simulink model "test1"  (R2020a)
settings: Solver=VariableStepAuto  StartTime=0.0  StopTime=inf  FixedStep=Ts  RelTol=1e-3
PostLoadFcn:
  | , if any(exist('dsrtsu_mdlpostloadfcn', 'file') ~= 0), dsrtsu_mdlpostloadfcn('Execute', bdroot); end,
InitFcn:
  | , if any(exist('rtifpga_mdlclblib', 'file') ~= 0), rtifpga_mdlclblib('Init', bdroot); end,
model workspace (MAT data in the model file):
  FPGA_test1_1_Interrupt_1_1_write : Simulink.Signal (value not decoded)
  FPGA_test1_1_Register_1_1_1_write : Simulink.Signal (value not decoded)
  FPGA_test1_1_Register_2_1_1_write : Simulink.Signal (value not decoded)
  FPGA_test1_1_Register_3_1_1_write : Simulink.Signal (value not decoded)
  FPGA_test1_1_Register_4_1_1_write : Simulink.Signal (value not decoded)
values from neighbouring files (symbols this model uses):
  clamp_threshold = 200    [param.m]
  io_fixed_gain = 10*1000/(3*100)    (= 33.3333333333)    [param.m]
  io_sonda_gain = 10/0.010    (= 1000)    [param.m]
  ioa_gain = 1    [param.m]
  ioa_offset = 0.12    [param.m]
  iob_gain = 1    [param.m]
  iob_offset = 0.06    [param.m]
  ioc_gain = 1    [param.m]
  ioc_offset = -0.1    [param.m]
  Ts = 20e-6    (= 2e-05)    [param.m]
  vclamp_gain = 1010    [param.m]
  vclamp_offset = 10.5    [param.m]
  vi_fixed_gain = 10*44    (= 440)    [param.m]
  vi_sonda_gain = 10*200    (= 2000)    [param.m]
  via_gain = 1    [param.m]
  via_offset = 2.2    [param.m]
  vib_gain = 1    [param.m]
  vib_offset = 3    [param.m]
  vic_gain = 1    [param.m]
  vic_offset = 4.2    [param.m]
libraries: xbsIndex_r4 x428, rti1202lib_adc_class1 x9, rtiproclib x6, simulink x2, rtifpgainterfacelib x1
(part 7 of 7)

== system test1/4_step/FPGA_IO_WRITE_BL6/dig_inout_tp1 ==
  note: The nominal input range is NOT simulated because
      | the HW does not saturate according to the input range.
  note: The Digital In value is simulated by Threshold voltage detection.
  data_in_i : Inport
  enable_i : Inport  Port=2
  data_out_i : Inport  Port=3
  direction_i : Inport  Port=4
  Data Type Conversion : DataTypeConversion
  Data Type Conversion1 : DataTypeConversion
  Disabled Input Value : Constant  Value=0
  Disabled Output Value : Constant  Value=0
  Invert : Constant  Value=inverted_dio
  Invert1 : Constant  Value=inverted_dio
  Inverter : Logic  Operator=NOT  AllPortsSameDT=off  OutDataTypeStr=boolean
  Inverter1 : Logic  AllPortsSameDT=off  OutDataTypeStr=boolean
  Inverter2 : Logic  Operator=NOT  AllPortsSameDT=off  OutDataTypeStr=boolean
  Inverter3 : Logic  AllPortsSameDT=off  OutDataTypeStr=boolean
  Inverter4 : Logic  Operator=NOT  AllPortsSameDT=off  OutDataTypeStr=boolean
  Relational Operator : RelationalOperator  OutDataTypeStr=boolean  RndMeth=Nearest
  Switch{,1..3} (4 alike) : Switch  Threshold=1
  Threshold Voltage : Constant  Value=2
  Voltage : Gain  Gain=voltage  ParamDataTypeStr=float('double')
  data_in_o : Outport  VectorParamsAs1DForOutWhenUnconnected=off
  data_out_o : Outport  Port=2  VectorParamsAs1DForOutWhenUnconnected=off
  wires:
  Voltage/1 -> data_out_o/1
  Data Type Conversion1/1 -> Inverter3/2, Inverter2/1
  Data Type Conversion/1 -> Inverter3/1, Inverter1/1
  Switch3/1 -> Voltage/1
  Switch2/1 -> Switch3/3, Inverter4/1
  Inverter4/1 -> Switch3/1
  Invert1/1 -> Switch3/2
  data_out_i/1 -> Switch2/1
  Inverter3/1 -> Switch2/2
  Disabled Output Value/1 -> Switch2/3
  Inverter2/1 -> Inverter1/2
  direction_i/1 -> Data Type Conversion1/1
  Inverter1/1 -> Switch/2
  enable_i/1 -> Data Type Conversion/1
  Switch/1 -> Switch1/3, Inverter/1
  Relational Operator/1 -> Switch/1
  Inverter/1 -> Switch1/1
  Invert/1 -> Switch1/2
  Switch1/1 -> data_in_o/1
  Disabled Input Value/1 -> Switch/3
  Threshold Voltage/1 -> Relational Operator/2
  data_in_i/1 -> Relational Operator/1

== system test1/4_step/FPGA_IO_WRITE_BL7/dig_inout_tp1 ==
  note: The nominal input range is NOT simulated because
      | the HW does not saturate according to the input range.
  note: The Digital In value is simulated by Threshold voltage detection.
  data_in_i : Inport
  enable_i : Inport  Port=2
  data_out_i : Inport  Port=3
  direction_i : Inport  Port=4
  Data Type Conversion : DataTypeConversion
  Data Type Conversion1 : DataTypeConversion
  Disabled Input Value : Constant  Value=0
  Disabled Output Value : Constant  Value=0
  Invert : Constant  Value=inverted_dio
  Invert1 : Constant  Value=inverted_dio
  Inverter : Logic  Operator=NOT  AllPortsSameDT=off  OutDataTypeStr=boolean
  Inverter1 : Logic  AllPortsSameDT=off  OutDataTypeStr=boolean
  Inverter2 : Logic  Operator=NOT  AllPortsSameDT=off  OutDataTypeStr=boolean
  Inverter3 : Logic  AllPortsSameDT=off  OutDataTypeStr=boolean
  Inverter4 : Logic  Operator=NOT  AllPortsSameDT=off  OutDataTypeStr=boolean
  Relational Operator : RelationalOperator  OutDataTypeStr=boolean  RndMeth=Nearest
  Switch{,1..3} (4 alike) : Switch  Threshold=1
  Threshold Voltage : Constant  Value=2
  Voltage : Gain  Gain=voltage  ParamDataTypeStr=float('double')
  data_in_o : Outport  VectorParamsAs1DForOutWhenUnconnected=off
  data_out_o : Outport  Port=2  VectorParamsAs1DForOutWhenUnconnected=off
  wires:
  Voltage/1 -> data_out_o/1
  Data Type Conversion1/1 -> Inverter3/2, Inverter2/1
  Data Type Conversion/1 -> Inverter3/1, Inverter1/1
  Switch3/1 -> Voltage/1
  Switch2/1 -> Switch3/3, Inverter4/1
  Inverter4/1 -> Switch3/1
  Invert1/1 -> Switch3/2
  data_out_i/1 -> Switch2/1
  Inverter3/1 -> Switch2/2
  Disabled Output Value/1 -> Switch2/3
  Inverter2/1 -> Inverter1/2
  direction_i/1 -> Data Type Conversion1/1
  Inverter1/1 -> Switch/2
  enable_i/1 -> Data Type Conversion/1
  Switch/1 -> Switch1/3, Inverter/1
  Relational Operator/1 -> Switch/1
  Inverter/1 -> Switch1/1
  Invert/1 -> Switch1/2
  Switch1/1 -> data_in_o/1
  Disabled Input Value/1 -> Switch/3
  Threshold Voltage/1 -> Relational Operator/2
  data_in_i/1 -> Relational Operator/1

== system test1/4_step/FPGA_IO_WRITE_BL8/dig_inout_tp1 ==
  note: The nominal input range is NOT simulated because
      | the HW does not saturate according to the input range.
  note: The Digital In value is simulated by Threshold voltage detection.
  data_in_i : Inport
  enable_i : Inport  Port=2
  data_out_i : Inport  Port=3
  direction_i : Inport  Port=4
  Data Type Conversion : DataTypeConversion
  Data Type Conversion1 : DataTypeConversion
  Disabled Input Value : Constant  Value=0
  Disabled Output Value : Constant  Value=0
  Invert : Constant  Value=inverted_dio
  Invert1 : Constant  Value=inverted_dio
  Inverter : Logic  Operator=NOT  AllPortsSameDT=off  OutDataTypeStr=boolean
  Inverter1 : Logic  AllPortsSameDT=off  OutDataTypeStr=boolean
  Inverter2 : Logic  Operator=NOT  AllPortsSameDT=off  OutDataTypeStr=boolean
  Inverter3 : Logic  AllPortsSameDT=off  OutDataTypeStr=boolean
  Inverter4 : Logic  Operator=NOT  AllPortsSameDT=off  OutDataTypeStr=boolean
  Relational Operator : RelationalOperator  OutDataTypeStr=boolean  RndMeth=Nearest
  Switch{,1..3} (4 alike) : Switch  Threshold=1
  Threshold Voltage : Constant  Value=2
  Voltage : Gain  Gain=voltage  ParamDataTypeStr=float('double')
  data_in_o : Outport  VectorParamsAs1DForOutWhenUnconnected=off
  data_out_o : Outport  Port=2  VectorParamsAs1DForOutWhenUnconnected=off
  wires:
  Voltage/1 -> data_out_o/1
  Data Type Conversion1/1 -> Inverter3/2, Inverter2/1
  Data Type Conversion/1 -> Inverter3/1, Inverter1/1
  Switch3/1 -> Voltage/1
  Switch2/1 -> Switch3/3, Inverter4/1
  Inverter4/1 -> Switch3/1
  Invert1/1 -> Switch3/2
  data_out_i/1 -> Switch2/1
  Inverter3/1 -> Switch2/2
  Disabled Output Value/1 -> Switch2/3
  Inverter2/1 -> Inverter1/2
  direction_i/1 -> Data Type Conversion1/1
  Inverter1/1 -> Switch/2
  enable_i/1 -> Data Type Conversion/1
  Switch/1 -> Switch1/3, Inverter/1
  Relational Operator/1 -> Switch/1
  Inverter/1 -> Switch1/1
  Invert/1 -> Switch1/2
  Switch1/1 -> data_in_o/1
  Disabled Input Value/1 -> Switch/3
  Threshold Voltage/1 -> Relational Operator/2
  data_in_i/1 -> Relational Operator/1

== system test1/4_step/FPGA_IO_WRITE_BL9/dig_inout_tp1 ==
  note: The nominal input range is NOT simulated because
      | the HW does not saturate according to the input range.
  note: The Digital In value is simulated by Threshold voltage detection.
  data_in_i : Inport
  enable_i : Inport  Port=2
  data_out_i : Inport  Port=3
  direction_i : Inport  Port=4
  Data Type Conversion : DataTypeConversion
  Data Type Conversion1 : DataTypeConversion
  Disabled Input Value : Constant  Value=0
  Disabled Output Value : Constant  Value=0
  Invert : Constant  Value=inverted_dio
  Invert1 : Constant  Value=inverted_dio
  Inverter : Logic  Operator=NOT  AllPortsSameDT=off  OutDataTypeStr=boolean
  Inverter1 : Logic  AllPortsSameDT=off  OutDataTypeStr=boolean
  Inverter2 : Logic  Operator=NOT  AllPortsSameDT=off  OutDataTypeStr=boolean
  Inverter3 : Logic  AllPortsSameDT=off  OutDataTypeStr=boolean
  Inverter4 : Logic  Operator=NOT  AllPortsSameDT=off  OutDataTypeStr=boolean
  Relational Operator : RelationalOperator  OutDataTypeStr=boolean  RndMeth=Nearest
  Switch{,1..3} (4 alike) : Switch  Threshold=1
  Threshold Voltage : Constant  Value=2
  Voltage : Gain  Gain=voltage  ParamDataTypeStr=float('double')
  data_in_o : Outport  VectorParamsAs1DForOutWhenUnconnected=off
  data_out_o : Outport  Port=2  VectorParamsAs1DForOutWhenUnconnected=off
  wires:
  Voltage/1 -> data_out_o/1
  Data Type Conversion1/1 -> Inverter3/2, Inverter2/1
  Data Type Conversion/1 -> Inverter3/1, Inverter1/1
  Switch3/1 -> Voltage/1
  Switch2/1 -> Switch3/3, Inverter4/1
  Inverter4/1 -> Switch3/1
  Invert1/1 -> Switch3/2
  data_out_i/1 -> Switch2/1
  Inverter3/1 -> Switch2/2
  Disabled Output Value/1 -> Switch2/3
  Inverter2/1 -> Inverter1/2
  direction_i/1 -> Data Type Conversion1/1
  Inverter1/1 -> Switch/2
  enable_i/1 -> Data Type Conversion/1
  Switch/1 -> Switch1/3, Inverter/1
  Relational Operator/1 -> Switch/1
  Inverter/1 -> Switch1/1
  Invert/1 -> Switch1/2
  Switch1/1 -> data_in_o/1
  Disabled Input Value/1 -> Switch/3
  Threshold Voltage/1 -> Relational Operator/2
  data_in_i/1 -> Relational Operator/1

== system test1/4_step/FPGA_XDATA_READ_BL1/phs_read_register ==
  note: Subsystem simulating the phs bus
      | access via RTLib functions.
  note: Subsystem simulating the communication
      | function specific behaviour. This is how the
      | FPGA framework driver takes effect on the data.
  data_i : Inport
  com_fct_model : Subsystem
  phs/rtlib_sim_model : Subsystem
  data_o : Outport  VectorParamsAs1DForOutWhenUnconnected=off
  data_new_o : Outport  Port=2  VectorParamsAs1DForOutWhenUnconnected=off
  wires:
  com_fct_model/2(data_new_o) -> data_new_o/1
  phs/rtlib_sim_model/1(data_o1) -> com_fct_model/1(data_i1)
  com_fct_model/1(data_o1) -> data_o/1
  data_i/1 -> phs/rtlib_sim_model/1(data_i1)

== system test1/4_step/FPGA_XDATA_READ_BL2/phs_read_register ==
  note: Subsystem simulating the phs bus
      | access via RTLib functions.
  note: Subsystem simulating the communication
      | function specific behaviour. This is how the
      | FPGA framework driver takes effect on the data.
  data_i : Inport
  com_fct_model : Subsystem
  phs/rtlib_sim_model : Subsystem
  data_o : Outport  VectorParamsAs1DForOutWhenUnconnected=off
  data_new_o : Outport  Port=2  VectorParamsAs1DForOutWhenUnconnected=off
  wires:
  com_fct_model/2(data_new_o) -> data_new_o/1
  phs/rtlib_sim_model/1(data_o1) -> com_fct_model/1(data_i1)
  com_fct_model/1(data_o1) -> data_o/1
  data_i/1 -> phs/rtlib_sim_model/1(data_i1)

== system test1/4_step/FPGA_XDATA_READ_BL3/phs_read_register ==
  note: Subsystem simulating the phs bus
      | access via RTLib functions.
  note: Subsystem simulating the communication
      | function specific behaviour. This is how the
      | FPGA framework driver takes effect on the data.
  data_i : Inport
  com_fct_model : Subsystem
  phs/rtlib_sim_model : Subsystem
  data_o : Outport  VectorParamsAs1DForOutWhenUnconnected=off
  data_new_o : Outport  Port=2  VectorParamsAs1DForOutWhenUnconnected=off
  wires:
  com_fct_model/2(data_new_o) -> data_new_o/1
  phs/rtlib_sim_model/1(data_o1) -> com_fct_model/1(data_i1)
  com_fct_model/1(data_o1) -> data_o/1
  data_i/1 -> phs/rtlib_sim_model/1(data_i1)

== system test1/4_step/FPGA_XDATA_READ_BL4/phs_read_register ==
  note: Subsystem simulating the phs bus
      | access via RTLib functions.
  note: Subsystem simulating the communication
      | function specific behaviour. This is how the
      | FPGA framework driver takes effect on the data.
  data_i : Inport
  com_fct_model : Subsystem
  phs/rtlib_sim_model : Subsystem
  data_o : Outport  VectorParamsAs1DForOutWhenUnconnected=off
  data_new_o : Outport  Port=2  VectorParamsAs1DForOutWhenUnconnected=off
  wires:
  com_fct_model/2(data_new_o) -> data_new_o/1
  phs/rtlib_sim_model/1(data_o1) -> com_fct_model/1(data_i1)
  com_fct_model/1(data_o1) -> data_o/1
  data_i/1 -> phs/rtlib_sim_model/1(data_i1)

== system test1/RTI Data/RTI Data Store/RTI Data Store ==
  RTI Data Store : Subsystem  mask(RTI_DATA_STORE){}
      mask help:
      | RTI Data Store Block. This block is used by RTI to store internal model dependent data. Deleting this block will result in data loss.
      |
      | NEVER DELETE, COPY, OR MODIFY THIS BLOCK!
      mask Help:
      | RTI Data Store Block. This block is used by RTI to store internal model dependent data. Deleting this block will result in data loss.
      | 
      | NEVER DELETE, COPY, OR MODIFY THIS BLOCK!
      mask Display: text(0.5, 0.5, ' ', 'HorizontalAlignment', 'center');

== system test1/4_step/FPGA_INT_BL1/phs_interrupt/com_fct_model ==
  data_i1 : Inport
  data_o1 : Outport  VectorParamsAs1DForOutWhenUnconnected=off
  wires:
  data_i1/1 -> data_o1/1

== system test1/4_step/FPGA_INT_BL1/phs_interrupt/phs//rtlib_sim_model ==
  note: - Detect the interrupt (rising edge).
      | - Generate function call.
  data_i1 : Inport
  Triggered Subsystem : Subsystem  TreatAsAtomicUnit=on
  data_o1 : Outport  VectorParamsAs1DForOutWhenUnconnected=off
  wires:
  Triggered Subsystem/1(Out1) -> data_o1/1
  data_i1/1 -> Triggered Subsystem/Trigger

== system test1/4_step/FPGA_XDATA_READ_BL1/phs_read_register/com_fct_model ==
  note: - Register data is presented to the FPGA application without data adaptions.
      |
      | - Register group accesses are implicitly simulated by simulink: all FPGA
      | communication function interface blocks are simulated within one task
      | with a unique sample time --> in- and ouputs are sampled simultaneously
      | and therefore data consistency is guaranteed.
  data_i1 : Inport
  Data_New_Calc : Subsystem
  Zero-Order Hold : ZeroOrderHold  SampleTime=fpga_sample_time
  data_o1 : Outport  VectorParamsAs1DForOutWhenUnconnected=off
  data_new_o : Outport  Port=2  VectorParamsAs1DForOutWhenUnconnected=off
  wires:
  Zero-Order Hold/1 -> data_o1/1
  Data_New_Calc/1(Out1) -> data_new_o/1
  data_i1/1 -> Zero-Order Hold/1, Data_New_Calc/1(In1)

== system test1/4_step/FPGA_XDATA_READ_BL1/phs_read_register/phs//rtlib_sim_model ==
  note: - The double to fixed-point conversion done by the XSG gateway behaves differently
      | than the conversion done by the RTLib C-code. Therefore the C-Code behaviour
      | is simulated via an s-function using the RTLib conversion technique including scaling and saturation.
  data_i1 : Inport
  S-Function : S-Function  FunctionName=DS1302_read_register  Parameters=mode;binaryPoint  SFunctionDeploymentMode=off  EnableBusSupport=off
  Zero-Order Hold : ZeroOrderHold  SampleTime=proc_sample_time
  data_o1 : Outport  VectorParamsAs1DForOutWhenUnconnected=off
  wires:
  Zero-Order Hold/1 -> S-Function/1
  S-Function/1 -> data_o1/1
  data_i1/1 -> Zero-Order Hold/1

== system test1/4_step/FPGA_XDATA_READ_BL2/phs_read_register/com_fct_model ==
  note: - Register data is presented to the FPGA application without data adaptions.
      |
      | - Register group accesses are implicitly simulated by simulink: all FPGA
      | communication function interface blocks are simulated within one task
      | with a unique sample time --> in- and ouputs are sampled simultaneously
      | and therefore data consistency is guaranteed.
  data_i1 : Inport
  Data_New_Calc : Subsystem
  Zero-Order Hold : ZeroOrderHold  SampleTime=fpga_sample_time
  data_o1 : Outport  VectorParamsAs1DForOutWhenUnconnected=off
  data_new_o : Outport  Port=2  VectorParamsAs1DForOutWhenUnconnected=off
  wires:
  Zero-Order Hold/1 -> data_o1/1
  Data_New_Calc/1(Out1) -> data_new_o/1
  data_i1/1 -> Zero-Order Hold/1, Data_New_Calc/1(In1)

== system test1/4_step/FPGA_XDATA_READ_BL2/phs_read_register/phs//rtlib_sim_model ==
  note: - The double to fixed-point conversion done by the XSG gateway behaves differently
      | than the conversion done by the RTLib C-code. Therefore the C-Code behaviour
      | is simulated via an s-function using the RTLib conversion technique including scaling and saturation.
  data_i1 : Inport
  S-Function : S-Function  FunctionName=DS1302_read_register  Parameters=mode;binaryPoint  SFunctionDeploymentMode=off  EnableBusSupport=off
  Zero-Order Hold : ZeroOrderHold  SampleTime=proc_sample_time
  data_o1 : Outport  VectorParamsAs1DForOutWhenUnconnected=off
  wires:
  Zero-Order Hold/1 -> S-Function/1
  S-Function/1 -> data_o1/1
  data_i1/1 -> Zero-Order Hold/1

== system test1/4_step/FPGA_XDATA_READ_BL3/phs_read_register/com_fct_model ==
  note: - Register data is presented to the FPGA application without data adaptions.
      |
      | - Register group accesses are implicitly simulated by simulink: all FPGA
      | communication function interface blocks are simulated within one task
      | with a unique sample time --> in- and ouputs are sampled simultaneously
      | and therefore data consistency is guaranteed.
  data_i1 : Inport
  Data_New_Calc : Subsystem
  Zero-Order Hold : ZeroOrderHold  SampleTime=fpga_sample_time
  data_o1 : Outport  VectorParamsAs1DForOutWhenUnconnected=off
  data_new_o : Outport  Port=2  VectorParamsAs1DForOutWhenUnconnected=off
  wires:
  Zero-Order Hold/1 -> data_o1/1
  Data_New_Calc/1(Out1) -> data_new_o/1
  data_i1/1 -> Zero-Order Hold/1, Data_New_Calc/1(In1)

== system test1/4_step/FPGA_XDATA_READ_BL3/phs_read_register/phs//rtlib_sim_model ==
  note: - The double to fixed-point conversion done by the XSG gateway behaves differently
      | than the conversion done by the RTLib C-code. Therefore the C-Code behaviour
      | is simulated via an s-function using the RTLib conversion technique including scaling and saturation.
  data_i1 : Inport
  S-Function : S-Function  FunctionName=DS1302_read_register  Parameters=mode;binaryPoint  SFunctionDeploymentMode=off  EnableBusSupport=off
  Zero-Order Hold : ZeroOrderHold  SampleTime=proc_sample_time
  data_o1 : Outport  VectorParamsAs1DForOutWhenUnconnected=off
  wires:
  Zero-Order Hold/1 -> S-Function/1
  S-Function/1 -> data_o1/1
  data_i1/1 -> Zero-Order Hold/1

== system test1/4_step/FPGA_XDATA_READ_BL4/phs_read_register/com_fct_model ==
  note: - Register data is presented to the FPGA application without data adaptions.
      |
      | - Register group accesses are implicitly simulated by simulink: all FPGA
      | communication function interface blocks are simulated within one task
      | with a unique sample time --> in- and ouputs are sampled simultaneously
      | and therefore data consistency is guaranteed.
  data_i1 : Inport
  Data_New_Calc : Subsystem
  Zero-Order Hold : ZeroOrderHold  SampleTime=fpga_sample_time
  data_o1 : Outport  VectorParamsAs1DForOutWhenUnconnected=off
  data_new_o : Outport  Port=2  VectorParamsAs1DForOutWhenUnconnected=off
  wires:
  Zero-Order Hold/1 -> data_o1/1
  Data_New_Calc/1(Out1) -> data_new_o/1
  data_i1/1 -> Zero-Order Hold/1, Data_New_Calc/1(In1)

== system test1/4_step/FPGA_XDATA_READ_BL4/phs_read_register/phs//rtlib_sim_model ==
  note: - The double to fixed-point conversion done by the XSG gateway behaves differently
      | than the conversion done by the RTLib C-code. Therefore the C-Code behaviour
      | is simulated via an s-function using the RTLib conversion technique including scaling and saturation.
  data_i1 : Inport
  S-Function : S-Function  FunctionName=DS1302_read_register  Parameters=mode;binaryPoint  SFunctionDeploymentMode=off  EnableBusSupport=off
  Zero-Order Hold : ZeroOrderHold  SampleTime=proc_sample_time
  data_o1 : Outport  VectorParamsAs1DForOutWhenUnconnected=off
  wires:
  Zero-Order Hold/1 -> S-Function/1
  S-Function/1 -> data_o1/1
  data_i1/1 -> Zero-Order Hold/1

== system test1/RTI Data/RTI Data Store/RTI Data Store/RTI Data Store ==
  RTI Data Store : Subsystem  mask(RTI_DATA_STORE){}
      mask help:
      | RTI Data Store Block. This block is used by RTI to store internal model dependent data. Deleting this block will result in data loss.
      |
      | NEVER DELETE, COPY, OR MODIFY THIS BLOCK!
      mask Help:
      | RTI Data Store Block. This block is used by RTI to store internal model dependent data. Deleting this block will result in data loss.
      | 
      | NEVER DELETE, COPY, OR MODIFY THIS BLOCK!
      mask Display: text(0.5, 0.5, ' ', 'HorizontalAlignment', 'center');

== system test1/4_step/FPGA_INT_BL1/phs_interrupt/phs//rtlib_sim_model/Triggered Subsystem ==
  Trigger : TriggerPort  VariantControl=(inherit)
  Function-Call Generator : simulink/Ports & Subsystems/Function-Call Generator  sample_time=-1  numberOfIterations=1
  Out1 : Outport  VectorParamsAs1DForOutWhenUnconnected=off
  wires:
  Function-Call Generator/1 -> Out1/1

== system test1/4_step/FPGA_XDATA_READ_BL1/phs_read_register/com_fct_model/Data_New_Calc ==
  note: The new data flag is presented whenever the input data port is sampled.
      | The flag is set to 1 for one FPGA simulation step and reset to 0 for the
      | remaining FPGA simulation steps contained within one processor simulation step.
  In1 : Inport
  Add : Sum
  Constant : Constant  Value=fpga_sample_time  SampleTime=fpga_sample_time
  Constant1 : Constant  Value=0
  Divide : Product  Inputs=*/
  Divide1 : Product  Inputs=*/
  Math Function : Math  Operator=mod  SignedPower=on  SaturateOnIntegerOverflow=on
  Relational Operator : RelationalOperator  Operator===  OutDataTypeStr=boolean  RndMeth=Nearest
  Unit Delay1 : UnitDelay  InitialCondition=-1  SampleTime=-1  HasFrameUpgradeWarning=on
  Weighted Sample Time1 : SampleTimeMath  TsampMathOp=Ts Only
  Out1 : Outport  VectorParamsAs1DForOutWhenUnconnected=off
  wires:
  Constant/1 -> Divide1/2, Divide1/1, Divide/2
  Weighted Sample Time1/1 -> Divide/1
  Math Function/1 -> Relational Operator/1
  Relational Operator/1 -> Out1/1
  In1/1 -> Weighted Sample Time1/1
  Divide1/1 -> Add/1
  Unit Delay1/1 -> Add/2
  Add/1 -> Unit Delay1/1, Math Function/1
  Constant1/1 -> Relational Operator/2
  Divide/1 -> Math Function/2

== system test1/4_step/FPGA_XDATA_READ_BL2/phs_read_register/com_fct_model/Data_New_Calc ==
  note: The new data flag is presented whenever the input data port is sampled.
      | The flag is set to 1 for one FPGA simulation step and reset to 0 for the
      | remaining FPGA simulation steps contained within one processor simulation step.
  In1 : Inport
  Add : Sum
  Constant : Constant  Value=fpga_sample_time  SampleTime=fpga_sample_time
  Constant1 : Constant  Value=0
  Divide : Product  Inputs=*/
  Divide1 : Product  Inputs=*/
  Math Function : Math  Operator=mod  SignedPower=on  SaturateOnIntegerOverflow=on
  Relational Operator : RelationalOperator  Operator===  OutDataTypeStr=boolean  RndMeth=Nearest
  Unit Delay1 : UnitDelay  InitialCondition=-1  SampleTime=-1  HasFrameUpgradeWarning=on
  Weighted Sample Time1 : SampleTimeMath  TsampMathOp=Ts Only
  Out1 : Outport  VectorParamsAs1DForOutWhenUnconnected=off
  wires:
  Constant/1 -> Divide1/2, Divide1/1, Divide/2
  Weighted Sample Time1/1 -> Divide/1
  Math Function/1 -> Relational Operator/1
  Relational Operator/1 -> Out1/1
  In1/1 -> Weighted Sample Time1/1
  Divide1/1 -> Add/1
  Unit Delay1/1 -> Add/2
  Add/1 -> Unit Delay1/1, Math Function/1
  Constant1/1 -> Relational Operator/2
  Divide/1 -> Math Function/2

== system test1/4_step/FPGA_XDATA_READ_BL3/phs_read_register/com_fct_model/Data_New_Calc ==
  note: The new data flag is presented whenever the input data port is sampled.
      | The flag is set to 1 for one FPGA simulation step and reset to 0 for the
      | remaining FPGA simulation steps contained within one processor simulation step.
  In1 : Inport
  Add : Sum
  Constant : Constant  Value=fpga_sample_time  SampleTime=fpga_sample_time
  Constant1 : Constant  Value=0
  Divide : Product  Inputs=*/
  Divide1 : Product  Inputs=*/
  Math Function : Math  Operator=mod  SignedPower=on  SaturateOnIntegerOverflow=on
  Relational Operator : RelationalOperator  Operator===  OutDataTypeStr=boolean  RndMeth=Nearest
  Unit Delay1 : UnitDelay  InitialCondition=-1  SampleTime=-1  HasFrameUpgradeWarning=on
  Weighted Sample Time1 : SampleTimeMath  TsampMathOp=Ts Only
  Out1 : Outport  VectorParamsAs1DForOutWhenUnconnected=off
  wires:
  Constant/1 -> Divide1/2, Divide1/1, Divide/2
  Weighted Sample Time1/1 -> Divide/1
  Math Function/1 -> Relational Operator/1
  Relational Operator/1 -> Out1/1
  In1/1 -> Weighted Sample Time1/1
  Divide1/1 -> Add/1
  Unit Delay1/1 -> Add/2
  Add/1 -> Unit Delay1/1, Math Function/1
  Constant1/1 -> Relational Operator/2
  Divide/1 -> Math Function/2

== system test1/4_step/FPGA_XDATA_READ_BL4/phs_read_register/com_fct_model/Data_New_Calc ==
  note: The new data flag is presented whenever the input data port is sampled.
      | The flag is set to 1 for one FPGA simulation step and reset to 0 for the
      | remaining FPGA simulation steps contained within one processor simulation step.
  In1 : Inport
  Add : Sum
  Constant : Constant  Value=fpga_sample_time  SampleTime=fpga_sample_time
  Constant1 : Constant  Value=0
  Divide : Product  Inputs=*/
  Divide1 : Product  Inputs=*/
  Math Function : Math  Operator=mod  SignedPower=on  SaturateOnIntegerOverflow=on
  Relational Operator : RelationalOperator  Operator===  OutDataTypeStr=boolean  RndMeth=Nearest
  Unit Delay1 : UnitDelay  InitialCondition=-1  SampleTime=-1  HasFrameUpgradeWarning=on
  Weighted Sample Time1 : SampleTimeMath  TsampMathOp=Ts Only
  Out1 : Outport  VectorParamsAs1DForOutWhenUnconnected=off
  wires:
  Constant/1 -> Divide1/2, Divide1/1, Divide/2
  Weighted Sample Time1/1 -> Divide/1
  Math Function/1 -> Relational Operator/1
  Relational Operator/1 -> Out1/1
  In1/1 -> Weighted Sample Time1/1
  Divide1/1 -> Add/1
  Unit Delay1/1 -> Add/2
  Add/1 -> Unit Delay1/1, Math Function/1
  Constant1/1 -> Relational Operator/2
  Divide/1 -> Math Function/2

== system test1/RTI Data/RTI Data Store/RTI Data Store/RTI Data Store/RTI Data Store ==

== matlab function test1/MATLAB Function1 ==
  data: u input; y output
function y = vector_to_ufix3(u)
y = 4*u(3) + 2*u(2) + u(1);

== matlab function test1/Subsystem/Function-Call Subsystem/MATLAB Function ==
  settings: updateMethod=DISCRETE
  data: iref input; y output; io input; vin input; T input
function y = fcn(iref, io, vin,T)
persistent kopt S
if(isempty(kopt))
    kopt = 19;
    S = [
     1 0 0 0 1 0 0 1 0; %+1
     0 1 0 1 0 0 1 0 0;
     0 1 0 0 0 1 0 0 1; %+2
     0 0 1 0 1 0 0 1 0;
     0 0 1 1 0 0 1 0 0; %+3
     1 0 0 0 0 1 0 0 1;
     0 1 0 1 0 0 0 1 0; %+4
     1 0 0 0 1 0 1 0 0;
     0 0 1 0 1 0 0 0 1; %+5
     0 1 0 0 0 1 0 1 0;
     1 0 0 0 0 1 1 0 0; %+6
     0 0 1 1 0 0 0 0 1;
     0 1 0 0 1 0 1 0 0; %+7
     1 0 0 1 0 0 0 1 0;
     0 0 1 0 0 1 0 1 0; %+8
     0 1 0 0 1 0 0 0 1;
     1 0 0 1 0 0 0 0 1; %+9
     0 0 1 0 0 1 1 0 0;
     1 0 0 1 0 0 1 0 0; %0A
     0 1 0 0 1 0 0 1 0; %0B
     0 0 1 0 0 1 0 0 1 %0C
     ];
end

fmin = inf;
R = 10;
L = 10e-3;

for k = 1:21
    v = [S(k,1:3); S(k,4:6); S(k,7:9)]*vin;
    ikk = (1-R*T/L)*io + T*v/L;
    e = iref - ikk;
    f = e'*e;
    if f < fmin
        fmin = f;
        kopt = k;
    end
end

y = kopt;
